simulink model "bungeeSimulink"  (R2014b)
settings: Solver=ode45  StartTime=0.0  StopTime=400  MaxStep=0.01  RelTol=1e-3
settings Model: Creator=malashy  LastModifiedBy=csimon

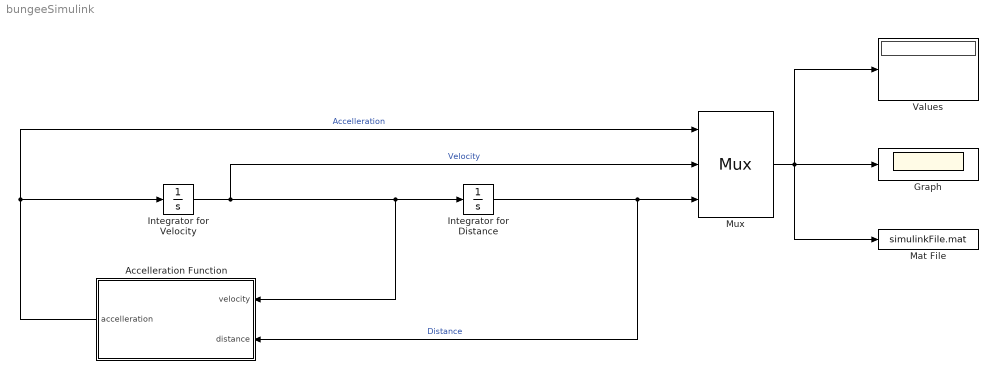
== system bungeeSimulink ==
  Accelleration Function : MATLAB Function  TreatAsAtomicUnit=on
  Graph : Scope
  Integrator for Distance : Integrator
  Integrator for Velocity : Integrator
  Mat File : ToFile  Filename=simulinkFile.mat  MatrixName=simulinkCalculation
  Mux : Mux  Inputs=3
      settings: DisplayOption=signals
  Values : Display
  wires:
  Integrator for Velocity/1 -> Accelleration Function/1(velocity), Integrator for Distance/1, Mux/2  "Velocity"
  Integrator for Distance/1 -> Accelleration Function/2(distance), Mux/3  "Distance"
  Mux/1 -> Mat File/1, Values/1, Graph/1
  Accelleration Function/1(accelleration) -> Mux/1, Integrator for Velocity/1  "Accelleration"

== matlab function bungeeSimulink/Accelleration Function ==
  data: velocity input; accelleration output; distance input
function accelleration = accelleration(velocity, distance)
    %{
        Returns the corresponding accelleration equation based on the input
        distance, x and the input velocity, dx
    %}
    if distance <= 100
        accelleration = (784.48 - 0.2502 .* (velocity .^ 2)) ./ 80;
    else
        accelleration = (784.48 - 0.2502 .* (velocity .^ 2) - 10 .* (distance - 100) - 1.5 .* velocity) / 80;
    end
end
